simulink model "pwm"  (R2022a)
settings: Solver=VariableStepAuto  StartTime=0.0  StopTime=0.1  RelTol=1e-3
values from neighbouring files (symbols this model uses):
  A = 1    [untitled.m]
  f = 50    [untitled.m]
  Pulse = 50    [untitled.m]
  pwm1_delay = 0    [untitled.m]
  pwm2_delay = T*(60/360)    (= 0.00333333333333)    [untitled.m]
  pwm3_delay = T*(120/360)    (= 0.00666666666667)    [untitled.m]
  pwm4_delay = T*(180/360)    (= 0.01)    [untitled.m]
  pwm5_delay = T*(-120/360)    (= -0.00666666666667)    [untitled.m]
  pwm6_delay = T*(-60/360)    (= -0.00333333333333)    [untitled.m]
  T = 1/f    (= 0.02)    [untitled.m]
  V_input = 550    [untitled.m]
libraries: spsIGBTDiodeLib x6, spsDCVoltageSourceLib x1, spsGroundLib x1, spsRMSLib x1, spsThreePhaseSeriesRLCBranchLib x1, spsThreePhaseVIMeasurementLib x1, spspowerguiLib x1
settings Model: Creator=hp  LastModifiedBy=hp

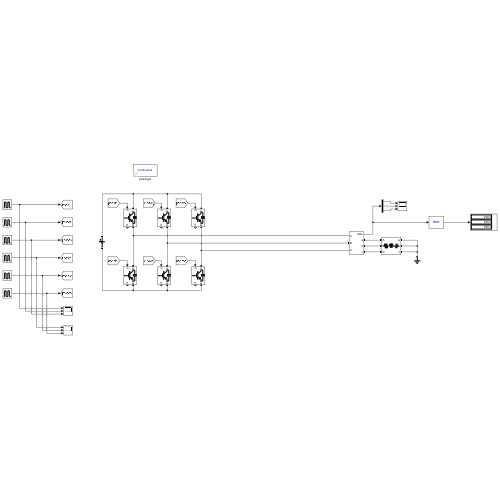
[thumbnail: Simulink's stored preview of the top-level diagram]
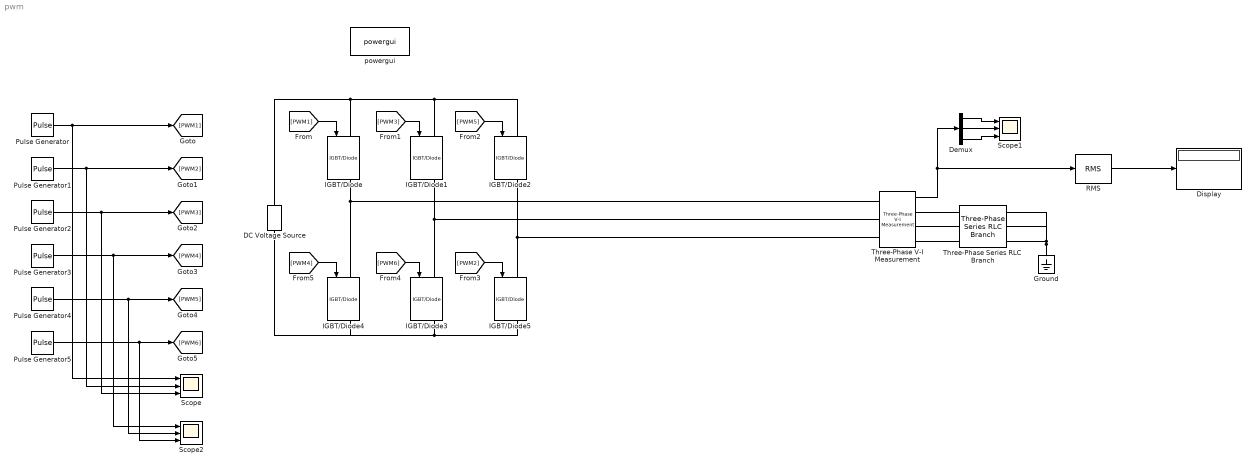
== system pwm ==
  DC Voltage Source : spsDCVoltageSourceLib/DC Voltage Source  Amplitude=V_input  Measurements=None
  Demux : Demux  Outputs=3
  Display : Display
  Ground : spsGroundLib/Ground  LConnTagsString=a
  IGBT/Diode{,1..5} (6 alike) : spsIGBTDiodeLib/IGBT//Diode  Ron=1e-3  Rs=1e5  Cs=inf  Measurements=on
  Pulse Generator : DiscretePulseGenerator  PulseType=Time based  Amplitude=A  Period=1/f  PulseWidth=Pulse  PhaseDelay=pwm1_delay
  Pulse Generator1 : DiscretePulseGenerator  PulseType=Time based  Amplitude=A  Period=T  PulseWidth=Pulse  PhaseDelay=pwm2_delay
  Pulse Generator2 : DiscretePulseGenerator  PulseType=Time based  Amplitude=A  Period=T  PulseWidth=Pulse  PhaseDelay=pwm3_delay
  Pulse Generator3 : DiscretePulseGenerator  PulseType=Time based  Amplitude=A  Period=T  PulseWidth=Pulse  PhaseDelay=pwm4_delay
  Pulse Generator4 : DiscretePulseGenerator  PulseType=Time based  Amplitude=A  Period=T  PulseWidth=Pulse  PhaseDelay=pwm5_delay
  Pulse Generator5 : DiscretePulseGenerator  PulseType=Time based  Amplitude=A  Period=T  PulseWidth=Pulse  PhaseDelay=pwm6_delay
  RMS : spsRMSLib/RMS  TrueRMS=on  Freq=f  RMSInit=1000  Ts=0
  Scope : Scope  NumInputPorts=3
  Scope1 : Scope  NumInputPorts=3
  Scope2 : Scope  NumInputPorts=3
  Three-Phase Series RLC Branch : spsThreePhaseSeriesRLCBranchLib/Three-Phase Series RLC Branch  LConnTagsString=A|B|C  RConnTagsString=A|B|C  BranchType=RLC  Resistance=1  Inductance=1e-3  Capacitance=1e-6  Measurements=None
  Three-Phase V-I Measurement : spsThreePhaseVIMeasurementLib/Three-Phase V-I Measurement  VoltageMeasurement=phase-to-ground  SetLabelV=off  LabelV=Vabc  Vpu=off  VpuLL=off  CurrentMeasurement=no  SetLabelI=off  LabelI=Iabc  Ipu=off  Pbase=100e6  Vbase=500e3  OutputType=Complex  PhasorSimulation=off  PSBequivalent=0
  powergui : spspowerguiLib/powergui  Priority=1  SimulationMode=Continuous  SampleTime=50e-6  frequency=60  Iterations=50  frequencyindice=0  Pbase=100e6  ErrMax=1e-4  UnitsV=kV  UnitsW=MW  buscounter=0  FunctionMessages=off  echomessages=off  EnableUseOfTLC=off  CurrentSourceSwitches=off  DisableSnubberDevices=off  DisableRonSwitches=off  DisableVfSwitches=off  DisplayEquations=off  AutomaticDiscreteSolvers=off  SolverType=Tustin/Backward Euler (TBE)  Interpol=off  ExternalGateDelay=off  methode=off  Ts=100  x0status=blocks  SPID=on  SwTol=0  HookPort=off  NonlinearTolerance=1e-4  nMaxIteration=100  ContinueOnMaxIteration=off  RestoreLinks=warning  ResistiveCurrentMeasurement=off  Frange=[0:2:500]  Ylog=off  Xlog=on  ShowGrid=off  save=off  variable=ZData  structure=0  ZoomFFT=off  StartTime=0.0  cycles=1  DisplayStyle=1  fundamental=60  FreqAxis=off  MaxFrequency=1000  frequencyindicesteady=1  RmsSteady=1  display=off
  wires:
  Three-Phase V-I Measurement/1 -> RMS/1, Demux/1
  Demux/3 -> Scope1/3
  Demux/2 -> Scope1/2
  [PWM3] -> IGBT/Diode1/1
  [PWM5] -> IGBT/Diode2/1
  [PWM6] -> IGBT/Diode3/1
  [PWM4] -> IGBT/Diode4/1
  [PWM2] -> IGBT/Diode5/1
  [PWM1] -> IGBT/Diode/1
  Demux/1 -> Scope1/1
  Pulse Generator/1 -> [PWM1], Scope/1
  Pulse Generator1/1 -> [PWM2], Scope/2
  Pulse Generator2/1 -> [PWM3], Scope/3
  Pulse Generator3/1 -> [PWM4], Scope2/1
  Pulse Generator4/1 -> Scope2/2, [PWM5]
  Pulse Generator5/1 -> [PWM6], Scope2/3
  RMS/1 -> Display/1
  connections:
  IGBT/Diode/RConn1 -- Three-Phase V-I Measurement/LConn1 -- IGBT/Diode4/LConn1
  IGBT/Diode2/LConn1 -- IGBT/Diode1/LConn1 -- DC Voltage Source/RConn1 -- IGBT/Diode/LConn1
  IGBT/Diode1/RConn1 -- Three-Phase V-I Measurement/LConn2 -- IGBT/Diode3/LConn1
  IGBT/Diode5/RConn1 -- IGBT/Diode4/RConn1 -- DC Voltage Source/LConn1 -- IGBT/Diode3/RConn1
  IGBT/Diode2/RConn1 -- Three-Phase V-I Measurement/LConn3 -- IGBT/Diode5/LConn1
  Ground/LConn1 -- Three-Phase Series RLC Branch/RConn3 -- Three-Phase Series RLC Branch/RConn1 -- Three-Phase Series RLC Branch/RConn2
  Three-Phase Series RLC Branch/LConn2 -- Three-Phase V-I Measurement/RConn2
  Three-Phase Series RLC Branch/LConn3 -- Three-Phase V-I Measurement/RConn3
  Three-Phase Series RLC Branch/LConn1 -- Three-Phase V-I Measurement/RConn1
